simulink model "pd_no_G_four"  (R2021a)
settings: Solver=VariableStepAuto  StartTime=0.0  StopTime=5  RelTol=1e-3
settings Model: Creator=Pouya  LastModifiedBy=lenovo
settings DebuggingCC: UnconnectedInputMsg=none  UnconnectedOutputMsg=none  UnconnectedLineMsg=none
settings ModelReferenceCC: EnableRefExpFcnMdlSchedulingChecks=off
settings RTWCC: Description=Generic Real-Time Target  DLArmComputeVersion=20.02.1

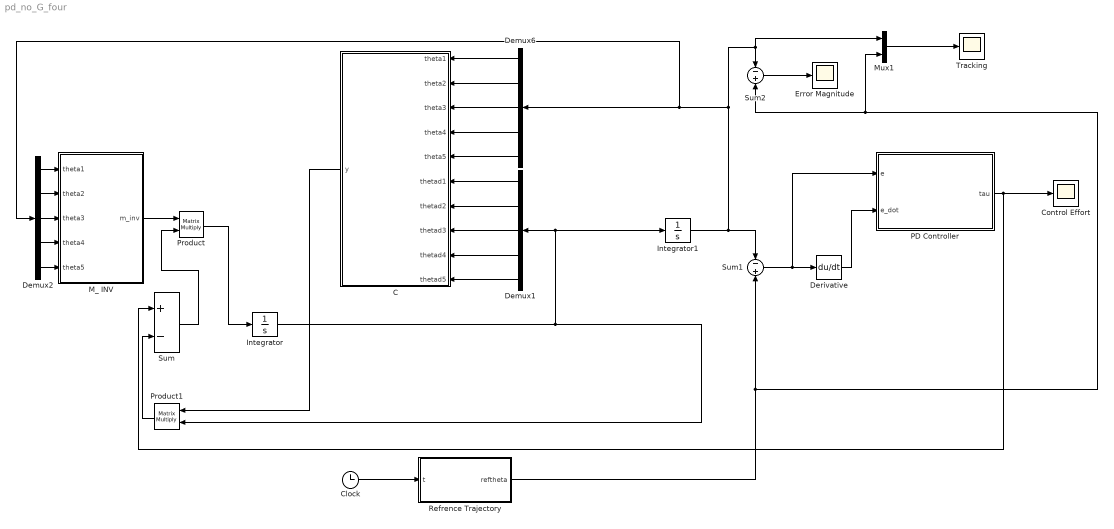
== system pd_no_G_four ==
  C : MATLAB Function  TreatAsAtomicUnit=on
  Clock : Clock
      settings: Decimation=5
  Control Effort : Scope
  Demux1 : Demux  Outputs=5
  Demux2 : Demux  Outputs=5
  Demux6 : Demux  Outputs=5
  Derivative : Derivative
  Error Magnitude : Scope
  Integrator : Integrator
  Integrator1 : Integrator
  M_ INV : MATLAB Function  TreatAsAtomicUnit=on
  Mux1 : Mux  Inputs=2
  PD Controller : MATLAB Function  TreatAsAtomicUnit=on
  Product : Product  Multiplication=Matrix(*)
  Product1 : Product  Multiplication=Matrix(*)
  Refrence Trajectory : MATLAB Function  TreatAsAtomicUnit=on
  Sum : Sum  Inputs=+-
  Sum1 : Sum  Inputs=-+
  Sum2 : Sum  Inputs=-+
  Tracking : Scope
  wires:
  PD Controller/1(tau) -> Sum/1, Control Effort/1
  Demux2/2 -> M_ INV/2(theta2)
  M_ INV/1(m_inv) -> Product/1
  Demux2/5 -> M_ INV/5(theta5)
  Demux2/4 -> M_ INV/4(theta4)
  C/1(y) -> Product1/1
  Demux2/3 -> M_ INV/3(theta3)
  Sum/1 -> Product/2
  Integrator/1 -> Demux1/1, Integrator1/1, Product1/2
  Product/1 -> Integrator/1
  Product1/1 -> Sum/2
  Demux2/1 -> M_ INV/1(theta1)
  Sum1/1 -> Derivative/1, PD Controller/1(e)
  Derivative/1 -> PD Controller/2(e_dot)
  Integrator1/1 -> Sum1/1, Demux2/1, Demux6/1, Mux1/1, Sum2/1
  Refrence Trajectory/1(reftheta) -> Mux1/2, Sum2/2, Sum1/2
  Sum2/1 -> Error Magnitude/1
  Mux1/1 -> Tracking/1
  Clock/1 -> Refrence Trajectory/1(t)
  Demux6/1 -> C/1(theta1)
  Demux6/2 -> C/2(theta2)
  Demux6/3 -> C/3(theta3)
  Demux6/4 -> C/4(theta4)
  Demux6/5 -> C/5(theta5)
  Demux1/1 -> C/6(thetad1)
  Demux1/2 -> C/7(thetad2)
  Demux1/3 -> C/8(thetad3)
  Demux1/4 -> C/9(thetad4)
  Demux1/5 -> C/10(thetad5)

== matlab function pd_no_G_four/C ==
  data: y output; theta1 input; theta2 input; theta3 input; theta4 input; theta5 input; thetad1 input; thetad2 input; thetad3 input; thetad4 input; thetad5 input
function y = C(theta1,theta2,theta3,theta4,theta5,thetad1,thetad2,thetad3,thetad4,thetad5)
C=zeros(5);
C(1,1) = 0.0000662161*thetad5 - 0.000132432*thetad5*cos(theta5)^2 - 0.0089*thetad3*cos(theta3) + 0.06345*thetad4*cos(theta4) - 0.91965*thetad3*sin(theta3) + 0.4185*thetad4*sin(theta4) + 0.06345*thetad3*cos(theta3)*cos(theta4) + 0.06345*thetad4*cos(theta3)*cos(theta4) + 0.4185*thetad3*cos(theta3)*sin(theta4) + 0.4185*thetad3*cos(theta4)*sin(theta3) + 0.4185*thetad4*cos(theta3)*sin(theta4) + 0.4185*thetad4*cos(theta4)*sin(theta3) + 0.00290548*thetad5*cos(theta5)*sin(theta5) - 0.06345*thetad3*sin(theta3)*sin(theta4) - 0.06345*thetad4*sin(theta3)*sin(theta4);
C(1,2) = 0.0000662161*thetad5 - 0.000132432*thetad5*cos(theta5)^2 - 0.00445*thetad3*cos(theta3) + 0.06345*thetad4*cos(theta4) - 0.459825*thetad3*sin(theta3) + 0.4185*thetad4*sin(theta4) + 0.031725*thetad3*cos(theta3)*cos(theta4) + 0.031725*thetad4*cos(theta3)*cos(theta4) + 0.20925*thetad3*cos(theta3)*sin(theta4) + 0.20925*thetad3*cos(theta4)*sin(theta3) + 0.20925*thetad4*cos(theta3)*sin(theta4) + 0.20925*thetad4*cos(theta4)*sin(theta3) + 0.00290548*thetad5*cos(theta5)*sin(theta5) - 0.031725*thetad3*sin(theta3)*sin(theta4) - 0.031725*thetad4*sin(theta3)*sin(theta4);
C(1,3) = 0.0000662161*thetad5 - 0.000132432*thetad5*cos(theta5)^2 - 0.0089*thetad1*cos(theta3) - 0.00445*thetad2*cos(theta3) - 0.0089*thetad3*cos(theta3) + 0.031725*thetad4*cos(theta4) - 0.91965*thetad1*sin(theta3) - 0.459825*thetad2*sin(theta3) - 0.16465*thetad3*sin(theta3) + 0.20925*thetad4*sin(theta4) + 0.06345*thetad1*cos(theta3)*cos(theta4) + 0.031725*thetad2*cos(theta3)*cos(theta4) + 0.06345*thetad3*cos(theta3)*cos(theta4) + 0.041025*thetad4*cos(theta3)*cos(theta4) + 0.4185*thetad1*cos(theta3)*sin(theta4) + 0.4185*thetad1*cos(theta4)*sin(theta3) + 0.20925*thetad2*cos(theta3)*sin(theta4) + 0.20925*thetad2*cos(theta4)*sin(theta3) + 0.4185*thetad3*cos(theta3)*sin(theta4) + 0.4185*thetad3*cos(theta4)*sin(theta3) + 0.20925*thetad4*cos(theta3)*sin(theta4) + 0.20925*thetad4*cos(theta4)*sin(theta3) + 0.00290548*thetad5*cos(theta5)*sin(theta5) - 0.06345*thetad1*sin(theta3)*sin(theta4) - 0.031725*thetad2*sin(theta3)*sin(theta4) - 0.06345*thetad3*sin(theta3)*sin(theta4) - 0.041025*thetad4*sin(theta3)*sin(theta4);
C(1,4) = 0.06345*thetad1*cos(theta4) + 0.06345*thetad2*cos(theta4) + 0.031725*thetad3*cos(theta4) + 0.0186*thetad4*cos(theta4) + 0.000218418*thetad5*cos(theta5) + 0.4185*thetad1*sin(theta4) + 0.4185*thetad2*sin(theta4) + 0.20925*thetad3*sin(theta4) + 0.00636181*thetad5*sin(theta5) + 0.06345*thetad1*cos(theta3)*cos(theta4) + 0.031725*thetad2*cos(theta3)*cos(theta4) + 0.041025*thetad3*cos(theta3)*cos(theta4) + 0.0186*thetad4*cos(theta3)*cos(theta4) + 0.4185*thetad1*cos(theta3)*sin(theta4) + 0.4185*thetad1*cos(theta4)*sin(theta3) + 0.20925*thetad2*cos(theta3)*sin(theta4) + 0.20925*thetad2*cos(theta4)*sin(theta3) + 0.20925*thetad3*cos(theta3)*sin(theta4) + 0.20925*thetad3*cos(theta4)*sin(theta3) - 0.06345*thetad1*sin(theta3)*sin(theta4) - 0.031725*thetad2*sin(theta3)*sin(theta4) - 0.041025*thetad3*sin(theta3)*sin(theta4) - 0.0186*thetad4*sin(theta3)*sin(theta4);
C(1,5) = 0.0000662161*thetad1 + 0.0000662161*thetad2 + 0.0000662161*thetad3 - 0.000132432*thetad1*cos(theta5)^2 - 0.000132432*thetad2*cos(theta5)^2 - 0.000132432*thetad3*cos(theta5)^2 + 0.000218418*thetad4*cos(theta5) + 0.000436835*thetad5*cos(theta5) + 0.00636181*thetad4*sin(theta5) + 0.0127236*thetad5*sin(theta5) + 0.00290548*thetad1*cos(theta5)*sin(theta5) + 0.00290548*thetad2*cos(theta5)*sin(theta5) + 0.00290548*thetad3*cos(theta5)*sin(theta5);
C(2,1) = 0.0000662161*thetad5 - 0.000132432*thetad5*cos(theta5)^2 - 0.00445*thetad3*cos(theta3) + 0.06345*thetad4*cos(theta4) - 0.459825*thetad3*sin(theta3) + 0.4185*thetad4*sin(theta4) + 0.031725*thetad3*cos(theta3)*cos(theta4) + 0.031725*thetad4*cos(theta3)*cos(theta4) + 0.20925*thetad3*cos(theta3)*sin(theta4) + 0.20925*thetad3*cos(theta4)*sin(theta3) + 0.20925*thetad4*cos(theta3)*sin(theta4) + 0.20925*thetad4*cos(theta4)*sin(theta3) + 0.00290548*thetad5*cos(theta5)*sin(theta5) - 0.031725*thetad3*sin(theta3)*sin(theta4) - 0.031725*thetad4*sin(theta3)*sin(theta4);
C(2,2) = 0.0000662161*thetad5 - 0.000132432*thetad5*cos(theta5)^2 + 0.06345*thetad4*cos(theta4) + 0.4185*thetad4*sin(theta4) + 0.00290548*thetad5*cos(theta5)*sin(theta5);
C(2,3) = 0.0000662161*thetad5 - 0.000132432*thetad5*cos(theta5)^2 - 0.00445*thetad1*cos(theta3) + 0.031725*thetad4*cos(theta4) - 0.459825*thetad1*sin(theta3) + 0.20925*thetad4*sin(theta4) + 0.031725*thetad1*cos(theta3)*cos(theta4) + 0.20925*thetad1*cos(theta3)*sin(theta4) + 0.20925*thetad1*cos(theta4)*sin(theta3) + 0.00290548*thetad5*cos(theta5)*sin(theta5) - 0.031725*thetad1*sin(theta3)*sin(theta4);
C(2,4) = 0.06345*thetad1*cos(theta4) + 0.06345*thetad2*cos(theta4) + 0.031725*thetad3*cos(theta4) + 0.0186*thetad4*cos(theta4) + 0.000218418*thetad5*cos(theta5) + 0.4185*thetad1*sin(theta4) + 0.4185*thetad2*sin(theta4) + 0.20925*thetad3*sin(theta4) + 0.00636181*thetad5*sin(theta5) + 0.031725*thetad1*cos(theta3)*cos(theta4) + 0.20925*thetad1*cos(theta3)*sin(theta4) + 0.20925*thetad1*cos(theta4)*sin(theta3) - 0.031725*thetad1*sin(theta3)*sin(theta4);
C(2,5) = 0.0000662161*thetad1 + 0.0000662161*thetad2 + 0.0000662161*thetad3 - 0.000132432*thetad1*cos(theta5)^2 - 0.000132432*thetad2*cos(theta5)^2 - 0.000132432*thetad3*cos(theta5)^2 + 0.000218418*thetad4*cos(theta5) + 0.000436835*thetad5*cos(theta5) + 0.00636181*thetad4*sin(theta5) + 0.0127236*thetad5*sin(theta5) + 0.00290548*thetad1*cos(theta5)*sin(theta5) + 0.00290548*thetad2*cos(theta5)*sin(theta5) + 0.00290548*thetad3*cos(theta5)*sin(theta5);
C(3,1) = 0.0000662161*thetad5 - 0.000132432*thetad5*cos(theta5)^2 + 0.0089*thetad1*cos(theta3) + 0.00445*thetad2*cos(theta3) + 0.031725*thetad4*cos(theta4) + 0.91965*thetad1*sin(theta3) + 0.459825*thetad2*sin(theta3) + 0.20925*thetad4*sin(theta4) - 0.06345*thetad1*cos(theta3)*cos(theta4) - 0.031725*thetad2*cos(theta3)*cos(theta4) + 0.022425*thetad4*cos(theta3)*cos(theta4) - 0.4185*thetad1*cos(theta3)*sin(theta4) - 0.4185*thetad1*cos(theta4)*sin(theta3) - 0.20925*thetad2*cos(theta3)*sin(theta4) - 0.20925*thetad2*cos(theta4)*sin(theta3) + 0.20925*thetad4*cos(theta3)*sin(theta4) + 0.20925*thetad4*cos(theta4)*sin(theta3) + 0.00290548*thetad5*cos(theta5)*sin(theta5) + 0.06345*thetad1*sin(theta3)*sin(theta4) + 0.031725*thetad2*sin(theta3)*sin(theta4) - 0.022425*thetad4*sin(theta3)*sin(theta4);
C(3,2) = 0.0000662161*thetad5 - 0.000132432*thetad5*cos(theta5)^2 + 0.00445*thetad1*cos(theta3) + 0.031725*thetad4*cos(theta4) + 0.459825*thetad1*sin(theta3) + 0.20925*thetad4*sin(theta4) - 0.031725*thetad1*cos(theta3)*cos(theta4) - 0.20925*thetad1*cos(theta3)*sin(theta4) - 0.20925*thetad1*cos(theta4)*sin(theta3) + 0.00290548*thetad5*cos(theta5)*sin(theta5) + 0.031725*thetad1*sin(theta3)*sin(theta4);
C(3,3) = 0.0000662161*thetad5 - 0.000132432*thetad5*cos(theta5)^2 + 0.00290548*thetad5*cos(theta5)*sin(theta5);
C(3,4) = 0.031725*thetad1*cos(theta4) + 0.031725*thetad2*cos(theta4) + 0.000218418*thetad5*cos(theta5) + 0.20925*thetad1*sin(theta4) + 0.20925*thetad2*sin(theta4) + 0.00636181*thetad5*sin(theta5) + 0.022425*thetad1*cos(theta3)*cos(theta4) + 0.20925*thetad1*cos(theta3)*sin(theta4) + 0.20925*thetad1*cos(theta4)*sin(theta3) - 0.022425*thetad1*sin(theta3)*sin(theta4);
C(3,5) = 0.0000662161*thetad1 + 0.0000662161*thetad2 + 0.0000662161*thetad3 - 0.000132432*thetad1*cos(theta5)^2 - 0.000132432*thetad2*cos(theta5)^2 - 0.000132432*thetad3*cos(theta5)^2 + 0.000218418*thetad4*cos(theta5) + 0.000436835*thetad5*cos(theta5) + 0.00636181*thetad4*sin(theta5) + 0.0127236*thetad5*sin(theta5) + 0.00290548*thetad1*cos(theta5)*sin(theta5) + 0.00290548*thetad2*cos(theta5)*sin(theta5) + 0.00290548*thetad3*cos(theta5)*sin(theta5);
C(4,1) = 0.000218418*thetad5*cos(theta5) - 0.06345*thetad2*cos(theta4) - 0.031725*thetad3*cos(theta4) - 0.06345*thetad1*cos(theta4) - 0.4185*thetad1*sin(theta4) - 0.4185*thetad2*sin(theta4) - 0.20925*thetad3*sin(theta4) + 0.00636181*thetad5*sin(theta5) - 0.06345*thetad1*cos(theta3)*cos(theta4) - 0.031725*thetad2*cos(theta3)*cos(theta4) - 0.022425*thetad3*cos(theta3)*cos(theta4) - 0.4185*thetad1*cos(theta3)*sin(theta4) - 0.4185*thetad1*cos(theta4)*sin(theta3) - 0.20925*thetad2*cos(theta3)*sin(theta4) - 0.20925*thetad2*cos(theta4)*sin(theta3) - 0.20925*thetad3*cos(theta3)*sin(theta4) - 0.20925*thetad3*cos(theta4)*sin(theta3) + 0.06345*thetad1*sin(theta3)*sin(theta4) + 0.031725*thetad2*sin(theta3)*sin(theta4) + 0.022425*thetad3*sin(theta3)*sin(theta4);
C(4,2) = 0.000218418*thetad5*cos(theta5) - 0.06345*thetad2*cos(theta4) - 0.031725*thetad3*cos(theta4) - 0.06345*thetad1*cos(theta4) - 0.4185*thetad1*sin(theta4) - 0.4185*thetad2*sin(theta4) - 0.20925*thetad3*sin(theta4) + 0.00636181*thetad5*sin(theta5) - 0.031725*thetad1*cos(theta3)*cos(theta4) - 0.20925*thetad1*cos(theta3)*sin(theta4) - 0.20925*thetad1*cos(theta4)*sin(theta3) + 0.031725*thetad1*sin(theta3)*sin(theta4);
C(4,3) = 0.000218418*thetad5*cos(theta5) - 0.031725*thetad2*cos(theta4) - 0.031725*thetad1*cos(theta4) - 0.20925*thetad1*sin(theta4) - 0.20925*thetad2*sin(theta4) + 0.00636181*thetad5*sin(theta5) - 0.022425*thetad1*cos(theta3)*cos(theta4) - 0.20925*thetad1*cos(theta3)*sin(theta4) - 0.20925*thetad1*cos(theta4)*sin(theta3) + 0.022425*thetad1*sin(theta3)*sin(theta4);
C(4,4) = 0.0;
C(4,5) = 0.000218418*thetad1*cos(theta5) + 0.000218418*thetad2*cos(theta5) + 0.000218418*thetad3*cos(theta5) + 0.00636181*thetad1*sin(theta5) + 0.00636181*thetad2*sin(theta5) + 0.00636181*thetad3*sin(theta5);
C(5,1) = 0.000132432*thetad1*cos(theta5)^2 - 0.0000662161*thetad2 - 0.0000662161*thetad3 - 0.0000662161*thetad1 + 0.000132432*thetad2*cos(theta5)^2 + 0.000132432*thetad3*cos(theta5)^2 - 0.000218418*thetad4*cos(theta5) - 0.00636181*thetad4*sin(theta5) - 0.00290548*thetad1*cos(theta5)*sin(theta5) - 0.00290548*thetad2*cos(theta5)*sin(theta5) - 0.00290548*thetad3*cos(theta5)*sin(theta5);
C(5,2) = 0.000132432*thetad1*cos(theta5)^2 - 0.0000662161*thetad2 - 0.0000662161*thetad3 - 0.0000662161*thetad1 + 0.000132432*thetad2*cos(theta5)^2 + 0.000132432*thetad3*cos(theta5)^2 - 0.000218418*thetad4*cos(theta5) - 0.00636181*thetad4*sin(theta5) - 0.00290548*thetad1*cos(theta5)*sin(theta5) - 0.00290548*thetad2*cos(theta5)*sin(theta5) - 0.00290548*thetad3*cos(theta5)*sin(theta5);
C(5,3) = 0.000132432*thetad1*cos(theta5)^2 - 0.0000662161*thetad2 - 0.0000662161*thetad3 - 0.0000662161*thetad1 + 0.000132432*thetad2*cos(theta5)^2 + 0.000132432*thetad3*cos(theta5)^2 - 0.000218418*thetad4*cos(theta5) - 0.00636181*thetad4*sin(theta5) - 0.00290548*thetad1*cos(theta5)*sin(theta5) - 0.00290548*thetad2*cos(theta5)*sin(theta5) - 0.00290548*thetad3*cos(theta5)*sin(theta5);
C(5,4) = - 0.000218418*thetad1*cos(theta5) - 0.000218418*thetad2*cos(theta5) - 0.000218418*thetad3*cos(theta5) - 0.00636181*thetad1*sin(theta5) - 0.00636181*thetad2*sin(theta5) - 0.00636181*thetad3*sin(theta5)
C(5,5) = 0.0;


y=C;

== matlab function pd_no_G_four/M_ INV ==
  data: theta1 input; m_inv output; theta2 input; theta3 input; theta4 input; theta5 input
function m_inv = M(theta1,theta2,theta3,theta4,theta5)
M=zeros(5);
M(1,1) = 1.8393*cos(theta3) - 0.837*cos(theta4) - 0.0178*sin(theta3) + 0.1269*sin(theta4) - 0.837*cos(theta3)*cos(theta4) + 0.1269*cos(theta3)*sin(theta4) + 0.1269*cos(theta4)*sin(theta3) - 0.000132432*cos(theta5)*sin(theta5) + 0.837*sin(theta3)*sin(theta4) - 0.00290548*cos(theta5)^2 + 3.61919;
M(1,2) = 0.91965*cos(theta3) - 0.837*cos(theta4) - 0.0089*sin(theta3) + 0.1269*sin(theta4) - 0.4185*cos(theta3)*cos(theta4) + 0.06345*cos(theta3)*sin(theta4) + 0.06345*cos(theta4)*sin(theta3) - 0.000132432*cos(theta5)*sin(theta5) + 0.4185*sin(theta3)*sin(theta4) - 0.00290548*cos(theta5)^2 + 2.35096;
M(1,3) = 0.16465*cos(theta3) - 0.4185*cos(theta4) - 0.0089*sin(theta3) + 0.06345*sin(theta4) - 0.4185*cos(theta3)*cos(theta4) + 0.06345*cos(theta3)*sin(theta4) + 0.06345*cos(theta4)*sin(theta3) - 0.000132432*cos(theta5)*sin(theta5) + 0.4185*sin(theta3)*sin(theta4) - 0.00290548*cos(theta5)^2 + 1.05864;
M(1,4) = 0.0186*sin(theta4) - 0.0127236*cos(theta5) + 0.000436835*sin(theta5) + 0.0186*cos(theta3)*sin(theta4) + 0.0186*cos(theta4)*sin(theta3) + 0.00328178;
M(1,5) = 0.000436835*sin(theta5) - 0.0127236*cos(theta5);
M(2,1) = 0.91965*cos(theta3) - 0.837*cos(theta4) - 0.0089*sin(theta3) + 0.1269*sin(theta4) - 0.4185*cos(theta3)*cos(theta4) + 0.06345*cos(theta3)*sin(theta4) + 0.06345*cos(theta4)*sin(theta3) - 0.000132432*cos(theta5)*sin(theta5) + 0.4185*sin(theta3)*sin(theta4) - 0.00290548*cos(theta5)^2 + 2.35096;
M(2,2) = 0.1269*sin(theta4) - 0.837*cos(theta4) - 0.000132432*cos(theta5)*sin(theta5) - 0.00290548*cos(theta5)^2 + 2.17141;
M(2,3) = 0.06345*sin(theta4) - 0.4185*cos(theta4) - 0.000132432*cos(theta5)*sin(theta5) - 0.00290548*cos(theta5)^2 + 1.05864;
M(2,4) = 0.0186*sin(theta4) - 0.0127236*cos(theta5) + 0.000436835*sin(theta5) + 0.00328178;
M(2,5) = 0.000436835*sin(theta5) - 0.0127236*cos(theta5);
M(3,1) = 0.16465*cos(theta3) - 0.4185*cos(theta4) - 0.0089*sin(theta3) + 0.06345*sin(theta4) - 0.4185*cos(theta3)*cos(theta4) + 0.06345*cos(theta3)*sin(theta4) + 0.06345*cos(theta4)*sin(theta3) - 0.000132432*cos(theta5)*sin(theta5) + 0.4185*sin(theta3)*sin(theta4) - 0.00290548*cos(theta5)^2 + 1.05864;
M(3,2) = 0.06345*sin(theta4) - 0.4185*cos(theta4) - 0.000132432*cos(theta5)*sin(theta5) - 0.00290548*cos(theta5)^2 + 1.05864;
M(3,3) = 0.893994 - 0.00290548*cos(theta5)^2 - 0.000132432*cos(theta5)*sin(theta5);
M(3,4) = 0.000436835*sin(theta5) - 0.0127236*cos(theta5) + 0.00328178;
M(3,5) = 0.000436835*sin(theta5) - 0.0127236*cos(theta5);
M(4,1) = 0.0186*sin(theta4) - 0.0127236*cos(theta5) + 0.000436835*sin(theta5) + 0.0186*cos(theta3)*sin(theta4) + 0.0186*cos(theta4)*sin(theta3) + 0.00328178;
M(4,2) = 0.0186*sin(theta4) - 0.0127236*cos(theta5) + 0.000436835*sin(theta5) + 0.00328178;
M(4,3) = 0.000436835*sin(theta5) - 0.0127236*cos(theta5) + 0.00328178;
M(4,4) = 0.551595;
M(4,5) = 0.00767374;
M(5,1) = 0.000436835*sin(theta5) - 0.0127236*cos(theta5);
M(5,2) = 0.000436835*sin(theta5) - 0.0127236*cos(theta5);
M(5,3) = 0.000436835*sin(theta5) - 0.0127236*cos(theta5);
M(5,4) = 0.00767374;
M(5,5) = 0.00767374;



m_inv =inv(M) ;

== matlab function pd_no_G_four/Refrence Trajectory ==
  data: t input; reftheta output
function reftheta  = Traj(t)
%reftheta = [0.5,0.5,0.5,0.5,0.5]';
%reftheta = [1,1,1,1,1]';
reftheta = [sin(0.5*t),sin(0.75*t),sin(t),sin(2.5*t),sin(3*t)]';
%reftheta = [sin(2*t),sin(2*t),sin(2*t),sin(2*t),sin(2*t)]';
end


% function reftheta = Traj(t)
%     % Define joint angles using smooth transitions
%     theta1 = 90 * smoothStep(t, 2, 3) - 90 * smoothStep(t, 4.1, 5);
%     theta2 = -50 * smoothStep(t, 0, 1) + 30 * smoothStep(t, 1.1, 2) ...
%              - 26 * smoothStep(t, 2, 3) + 46 * smoothStep(t, 3.1, 5);
%     theta3 = 20 * smoothStep(t, 0, 1) - 8 * smoothStep(t, 1.1, 2) ...
%              - 12 * smoothStep(t, 3.1, 5);
%     theta4 = -43 * smoothStep(t, 0, 1) + 5 * smoothStep(t, 1.1, 2) ...
%              + 38 * smoothStep(t, 3.1, 5);
%     theta5 = 90 * smoothStep(t, 0, 1) - 90 * smoothStep(t, 4.1, 5);
% 
%     % Return the angles in a column vector
%     reftheta = [theta1, theta2, theta3, theta4, theta5]';
% end
% function y = smoothStep(t, t0, t1)
%     if t <= t0
%         y = 0;
%     elseif t >= t1
%         y = 1;
%     else
%         y = (t - t0) / (t1 - t0);
%     end
% end

== matlab function pd_no_G_four/PD Controller ==
  data: e input; tau output; e_dot input
function tau = PD_controller(e,e_dot)
kp =[70    0     0     0     0 ;
     0     70    0     0     0 ;
     0     0     70    0     0 ;
     0     0     0     50    0 ;
     0     0     0     0     50];

kd =[40   0      0      0     0 ;
     0    40     0      0     0 ;
     0     0     30     0     0 ;
     0     0     0     20     0 ;
     0     0     0      0    10 ];
tau = kp*e + kd*e_dot;
